simulink model "simplest6_noMPC"  (Simulink 7.4)
settings: Solver=FixedStepDiscrete  StartTime=0.0  StopTime=inf  RelTol=1e-3
PreLoadFcn:
  | RTWConfigurationCB('preloadfcn', bdroot);
PostLoadFcn:
  | mpc555rt_switch_target(gcs,'auto')
CloseFcn:
  | rtwprivate ssgencode ModelCloseRequest foo
settings Model: Creator=The MathWorks Inc.  LastModifiedBy=autopilot
settings DataIOCC: LimitDataPoints=off  SignalLoggingName=sigsOut
settings OptimizationCC: InlineParams=on  InlineInvariantSignals=on  EnforceIntegerDowncast=off  ZeroExternalMemoryAtStartup=off  ZeroInternalMemoryAtStartup=off  InitFltsAndDblsToZero=on  NoFixptDivByZeroProtection=on  OptimizeModelRefInitCode=on  LifeSpan=1
settings DebuggingCC: SaveWithParameterizedLinksMsg=none  SignalResolutionControl=TryResolveAllWithWarning  SolverPrmCheckMsg=none  MultiTaskDSMMsg=warning  MultiTaskCondExecSysMsg=none  UnderSpecifiedDataTypeMsg=error  StrictBusMsg=None
settings HardwareCC: ProdEndianess=BigEndian  ProdHWDeviceType=Motorola PowerPC
settings RTWCC: SystemTargetFile=mpc555rt.tlc  TemplateMakefile=mpc555rt.tmf  Description=Target Support Package (for use with Freescale MPC5xx) (real-time)  ProcessScript=mpc555rt_make_rtw_hook
settings CodeAppCC: IgnoreCustomStorageClasses=off
settings STFCustomTargetCC: TargetFcnLib=ansi_tfl_tmw.mat  TargetLibSuffix=.a  TargetPreCompLibLocation=C:\Program Files\MATLAB\R2009b\toolbox\rtw\targets\mpc555dk\drivers\lib\DIAB  IncludeMdlTerminateFcn=off  CombineOutputUpdateFcns=on  ERTCustomFileBanners=on  SupportAbsoluteTime=off  SupportNonFinite=off  SupportComplex=off  SupportContinuousTime=off  SupportNonInlinedSFcns=off  CPPClassGenCompliant=on  SystemTargetFile=mpc555rt.tlc
settings ERTTargetCC: TargetFcnLib=ansi_tfl_tmw.mat  TargetPreCompLibLocation=C:\Program Files\MATLAB\R2009b\toolbox\rtw\targets\mpc555dk\drivers\lib\DIAB  MultiwordLength=2048  ParMdlRefBuildCompliant=off  CompOptLevelCompliant=off  IncludeMdlTerminateFcn=off  ERTFirstTimeCompliant=off  SupportAbsoluteTime=off  SupportNonFinite=off  SupportComplex=off  ModelStepFunctionPrototypeControlCompliant=off  ExtModeMexFile=MPC5xxExternalModeOpen  ExtModeIntrfLevel=Level2 - Open  ERTCustomFileTemplate=example_file_process.tlc  ConvertIfToSwitch=off
settings CustomProperty: DataType=RTWOptions_EnumType__toolbox_rtw_targets_mpc555dk_mpc555dk_mpc555rt_1MPC555_OPTIMIZATION_SWITCH  Value=speed
settings EnumStrPairs: String=speed

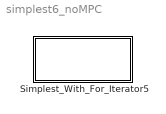
== system simplest6_noMPC ==
  Simplest_With_For_Iterator5 : Subsystem  TreatAsAtomicUnit=on

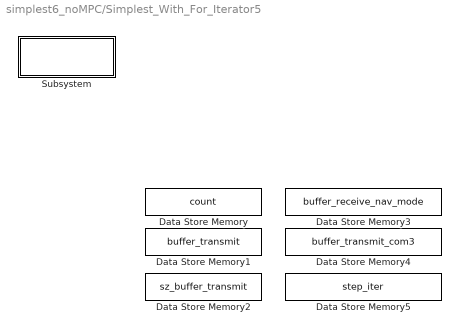
== system simplest6_noMPC/Simplest_With_For_Iterator5 ==
  Data Store Memory : DataStoreMemory  DataStoreName=count  DataType=uint8  OutDataType=fixdt(1, 16)  OutScaling=2^0  OutDataTypeStr=uint8
  Data Store Memory1 : DataStoreMemory  DataStoreName=buffer_transmit  InitialValue=[0 0 0 0 0 0 0 0 0 0 0]  DataType=uint8  OutDataType=fixdt(1, 16)  OutScaling=2^0  OutDataTypeStr=uint8
  Data Store Memory2 : DataStoreMemory  DataStoreName=sz_buffer_transmit  DataType=uint32  OutDataType=fixdt(1, 16)  OutScaling=2^0  OutDataTypeStr=uint32
  Data Store Memory3 : DataStoreMemory  DataStoreName=buffer_receive_nav_mode  InitialValue=[0 0 0 0 0 0 0 0 0 0 0 0 0 0 0 0 0 0 0 0 0 0 0 0 0 0 0 0 0 0 0 0 0 0 0 0 0]  DataType=uint8  OutDataType=fixdt(1, 16)  OutScaling=2^0  OutDataTypeStr=uint8
  Data Store Memory4 : DataStoreMemory  DataStoreName=buffer_transmit_com3  InitialValue=[65 66 67 68 69 70 71 72 73 74 75 76 77 78 79 13 10]  DataType=uint8  OutDataType=fixdt(1, 16)  OutScaling=2^0  OutDataTypeStr=uint8
  Data Store Memory5 : DataStoreMemory  DataStoreName=step_iter  DataType=uint8  OutDataType=fixdt(1, 16)  OutScaling=2^0  OutDataTypeStr=uint8
  Subsystem : Subsystem  TreatAsAtomicUnit=on

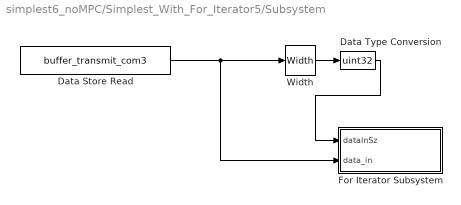
== system simplest6_noMPC/Simplest_With_For_Iterator5/Subsystem ==
  Data Store Read : DataStoreRead  DataStoreName=buffer_transmit_com3  SampleTime=-1
  Data Type Conversion : DataTypeConversion  OutDataTypeMode=uint32  OutDataType=fixdt(1, 16)  OutScaling=2^0  OutDataTypeStr=uint32
  For Iterator Subsystem : Subsystem  TreatAsAtomicUnit=on
  Width : Width
  wires:
  Data Store Read/1 -> Width/1, For Iterator Subsystem/2(data_in)
  Width/1 -> Data Type Conversion/1
  Data Type Conversion/1 -> For Iterator Subsystem/1(dataInSz)

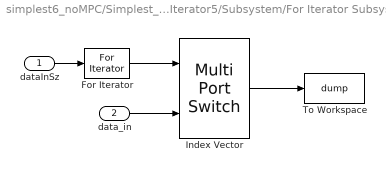
== system simplest6_noMPC/Simplest_With_For_Iterator5/Subsystem/For Iterator Subsystem ==
  dataInSz : Inport  DataType=uint32  OutDataType=fixdt(1, 16)  OutScaling=2^0  OutDataTypeStr=uint32
  data_in : Inport  Port=2  DataType=uint8  OutDataType=fixdt(1, 16)  OutScaling=2^0  OutDataTypeStr=uint8
  For Iterator : ForIterator  IterationSource=external
  Index Vector : MultiPortSwitch  Inputs=1  OutDataType=fixdt(1, 16)  OutScaling=2^0
  To Workspace : ToWorkspace  VariableName=dump  SampleTime=-1  SaveFormat=Structure
  wires:
  dataInSz/1 -> For Iterator/1
  For Iterator/1 -> Index Vector/1
  data_in/1 -> Index Vector/2
  Index Vector/1 -> To Workspace/1
